simulink model "atthw9"  (R2018b)
settings: Solver=VariableStepAuto  StartTime=0.0  StopTime=6000  RelTol=1e-3
settings Model: Creator=Eric  LastModifiedBy=Eric

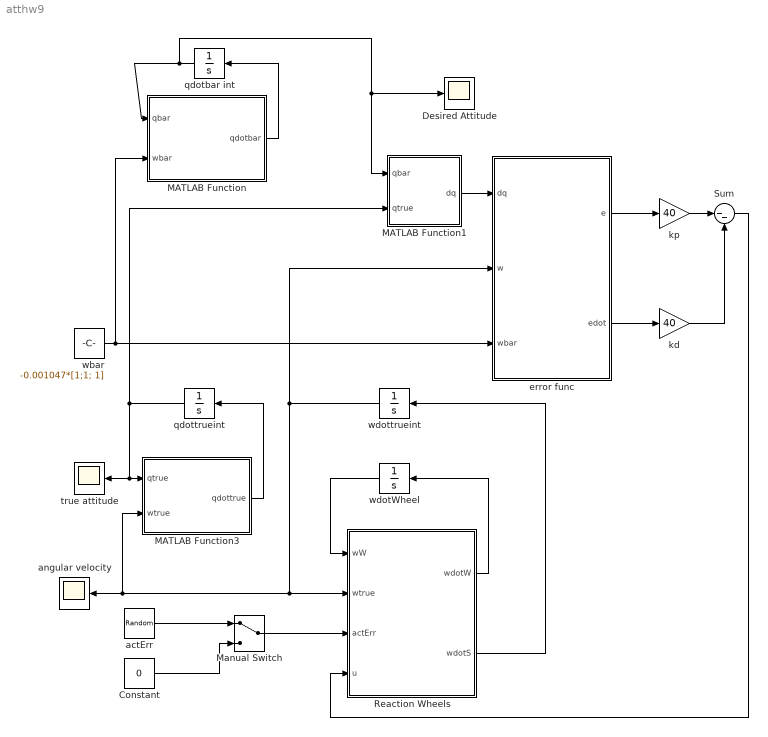
== system atthw9 ==
  Constant : Constant  Value=0
  Desired Attitude : Scope
  MATLAB Function : MATLAB Function  TreatAsAtomicUnit=on
  MATLAB Function1 : MATLAB Function  TreatAsAtomicUnit=on
  MATLAB Function3 : MATLAB Function  TreatAsAtomicUnit=on
  Manual Switch : ManualSwitch
  "Reaction Wheels " : MATLAB Function  TreatAsAtomicUnit=on
  Sum : Sum  Inputs=|--
  actErr : RandomNumber  Variance=20  SampleTime=0.1
  angular velocity : Scope
  error func : MATLAB Function  TreatAsAtomicUnit=on
  kd : Gain  Gain=40
  kp : Gain  Gain=40
  qdotbar int : Integrator  InitialCondition=[ .5; .5; .5; .5]
  qdottrueint : Integrator  InitialCondition=[ .491;.491;.509;.509]/norm([ .491;.491;.509;.509])
  true attitude : Scope
  "wbar " : Constant  Value=-0.001047*[1;1; 1]  OutDataTypeStr=Inherit: Inherit via back propagation
  wdotWheel : Integrator  InitialCondition=[6.92;6.92;6.92]
  wdottrueint : Integrator  InitialCondition=[.01; 0; 0]
  wires:
  "wbar "/1 -> MATLAB Function/2(wbar), error func/3(wbar)
  MATLAB Function1/1(dq) -> error func/1(dq)
  MATLAB Function3/1(qdottrue) -> qdottrueint/1
  qdottrueint/1 -> MATLAB Function3/1(qtrue), true attitude/1, MATLAB Function1/2(qtrue)
  wdottrueint/1 -> error func/2(w), "Reaction Wheels "/2(wtrue), MATLAB Function3/2(wtrue), angular velocity/1
  error func/1(e) -> kp/1
  error func/2(edot) -> kd/1
  kp/1 -> Sum/1
  kd/1 -> Sum/2
  qdotbar int/1 -> MATLAB Function1/1(qbar), Desired Attitude/1, MATLAB Function/1(qbar)
  MATLAB Function/1(qdotbar) -> qdotbar int/1
  "Reaction Wheels "/2(wdotS) -> wdottrueint/1
  "Reaction Wheels "/1(wdotW) -> wdotWheel/1
  wdotWheel/1 -> "Reaction Wheels "/1(wW)
  Sum/1 -> "Reaction Wheels "/4(u)
  Manual Switch/1 -> "Reaction Wheels "/3(actErr)
  actErr/1 -> Manual Switch/1
  Constant/1 -> Manual Switch/2

== matlab function atthw9/MATLAB Function1 ==
  data: qbar input; dq output; qtrue input
function dq = dq(qbar,qtrue)
qbar(2:4) = -qbar(2:4);
dq = quatMult(qtrue, qbar);

== matlab function atthw9/MATLAB Function ==
  data: qbar input; qdotbar output; wbar input
function qdotbar = qdotbar(qbar,wbar)
qwbar = .5*[0; wbar];
qdotbar = quatMult(qbar, qwbar);

== matlab function atthw9/error func ==
  data: dq input; e output; w input; wbar input; edot output
function [e, edot] = error(dq, w, wbar)

%2
e = 2*(dq(2:4)/dq(1));

%3
dw = w - wbar;
wbskew = [0, -w(3), w(2); w(3), 0, -w(1); -w(2), w(1), 0]; 
edot = -wbskew*e + dw;

== matlab function atthw9/MATLAB Function3 ==
  data: qtrue input; qdottrue output; wtrue input
function qdottrue = qdottrue(qtrue, wtrue)
qwtrue = [0; wtrue];
qdottrue = .5*quatMult(qwtrue, qtrue);

== matlab function atthw9/Reaction Wheels  ==
  data: wW input; wdotW output; wtrue input; actErr input; u input; wdotS output
function [wdotW, wdotS]    = reactionWheels(wW, wtrue, actErr, u)

%reaction wheel specs
%http://bluecanyontech.com/rw4/
mw = 3; %kg
r = .17; %m
h = .07; %m
A = (1/12)*mw*(3*r^2 + h^2); 
C = .5*mw*r^2;
Jw1 = [A, 0, 0; 0, A, 0; 0, 0, C];
Jw2 = [A, 0, 0; 0, C, 0; 0, 0, A];
Jw3 = [C, 0, 0; 0, A, 0; 0, 0, A];

% %inertia tensor of spacecraft
JcgB = [1000, 0, 0; 0, 500, 0; 0, 0, 600];
lskew = [0,-1,1;1,0,-1;-1,1,0];  %[m]. Each wheel is located along 1 meter along a body axis
JcgS = JcgB + Jw1 + Jw2 *Jw3 - 3*mw*lskew^2;
wdotW = -cross(wtrue, wW) - u - actErr;
wdotS = inv(JcgS)*(-cross(wtrue,JcgB*wtrue) - C*wdotW - cross(wtrue,C*wW));
